simulink model "feedback_example"  (Simulink 7.5)
settings: Solver=ode45  StartTime=0.0  StopTime=10.0  RelTol=1e-3
undefined symbols (not defined in the file): kI
settings Model: Creator=jporter  LastModifiedBy=jporter

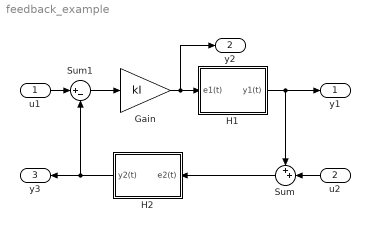
== system feedback_example ==
  u1 : Inport  OutDataType=fixdt(1, 16)  OutScaling=2^0
  u2 : Inport  Port=2  OutDataType=fixdt(1, 16)  OutScaling=2^0
  Gain : Gain  Gain=kI  ParameterDataType=fixdt(1, 16)  ParameterScaling=2^0  OutDataType=fixdt(1, 16)  OutScaling=2^0
  H1 : Subsystem
  H2 : Subsystem
  Sum : Sum  Inputs=++|  OutDataType=fixdt(1, 16)  OutScaling=2^0
  Sum1 : Sum  Inputs=|+-  OutDataType=fixdt(1, 16)  OutScaling=2^0
  y1 : Outport  OutDataType=fixdt(1, 16)  OutScaling=2^0
  y2 : Outport  Port=2  OutDataType=fixdt(1, 16)  OutScaling=2^0
  y3 : Outport  Port=3  OutDataType=fixdt(1, 16)  OutScaling=2^0
  wires:
  u1/1 -> Sum1/1
  Sum1/1 -> Gain/1
  Gain/1 -> H1/1(e1(t)), y2/1
  H1/1(y1(t)) -> y1/1, Sum/1
  u2/1 -> Sum/2
  Sum/1 -> H2/1(e2(t))
  H2/1(y2(t)) -> Sum1/2, y3/1

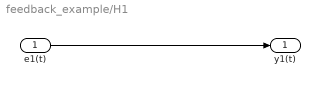
== system feedback_example/H1 ==
  e1(t) : Inport  OutDataType=fixdt(1, 16)  OutScaling=2^0
  y1(t) : Outport  OutDataType=fixdt(1, 16)  OutScaling=2^0
  wires:
  e1(t)/1 -> y1(t)/1

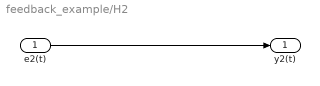
== system feedback_example/H2 ==
  e2(t) : Inport  OutDataType=fixdt(1, 16)  OutScaling=2^0
  y2(t) : Outport  OutDataType=fixdt(1, 16)  OutScaling=2^0
  wires:
  e2(t)/1 -> y2(t)/1
